simulink library "relay_housing_lib"  (Simulink 8.1)
settings: Solver=ode45  StartTime=0.0  StopTime=10.0  RelTol=1e-3
undefined symbols (not defined in the file): F0, F1, F2, F3, F4, Ts
libraries: relay_modbus_lib x137, rtio_generic_modbus x69, rtlab x10, simulink_extras x10, simulink x6, RMS_lib x4, relay_PLL_lib x3, powerlib_extras x2, relay_ANSI_functions_lib x2, relay_PQSPF_lib x1, powerlib_meascontrol x1, relay_mgc_cmd_lib x1
(part 1 of 3)
settings Model: Creator=re25624  LastModifiedBy=hptb1

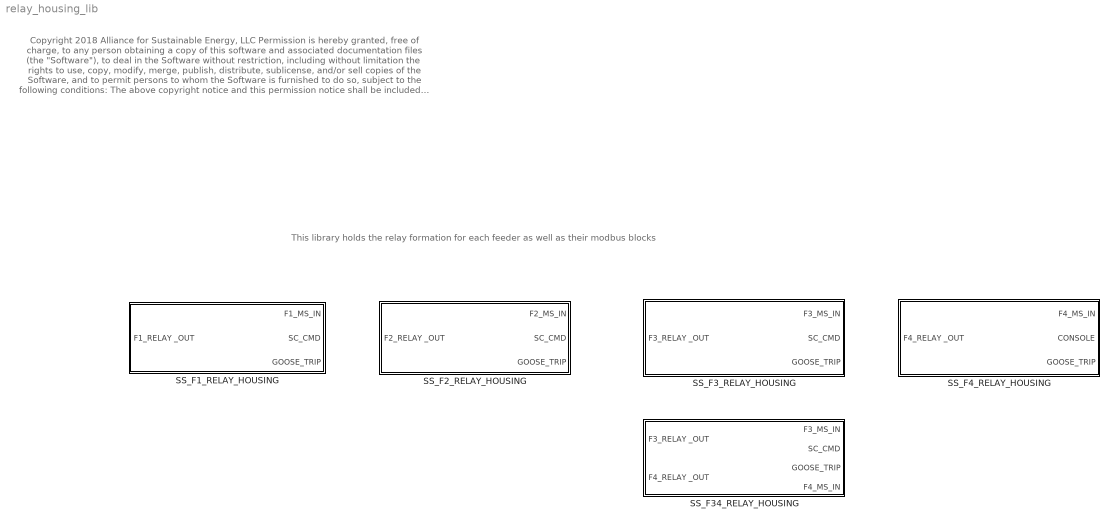
== system relay_housing_lib ==
  note: This library holds the relay formation for each feeder as well as their modbus blocks
  note: Copyright 2018 Alliance for Sustainable Energy, LLC
      |
      | Permission is hereby granted, free of charge, to any person obtaining a copy of this software
      | and associated documentation files (the "Software"), to deal in the Software without restriction,
      | including without limitation the rights to use, copy, modify, merge, publish, distribute, sublicense,
      | and/or sell copies of the Software, and to permit persons to whom the Software is furnished to do so,
      | subject to the following conditions:
      |
      | The above copyright notice and this permission notice shall be included in all copies or substantial portions of the Software.
      |
      | THE SOFTWARE IS PROVIDED "AS IS", WITHOUT WARRANTY OF ANY KIND, EXPRESS OR IMPLIED, INCLUDING
      | BUT NOT LIMITED TO THE WARRANTIES OF MERCHANTABILITY, FITNESS FOR A PARTICULAR PURPOSE AND
      | NONINFRINGEMENT. IN NO EVENT SHALL THE AUTHORS, THE COPYRIGHT HOLDERS, THE UNITED STATES,
      | THE UNITED STATES DEPARTMENT OF ENERGY, OR ANY OF THEIR EMPLOYEES BE LIABLE FOR ANY CLAIM,
      | DAMAGES OR OTHER LIABILITY, WHETHER IN AN ACTION OF CONTRACT, TORT OR OTHERWISE, ARISING FROM,
      | OUT OF OR IN CONNECTION WITH THE SOFTWARE OR THE USE OR OTHER DEALINGS IN THE SOFTWARE.
  SS_F1_RELAY_HOUSING : Subsystem
  SS_F2_RELAY_HOUSING : Subsystem
  SS_F34_RELAY_HOUSING : Subsystem
  SS_F3_RELAY_HOUSING : Subsystem
  SS_F4_RELAY_HOUSING : Subsystem

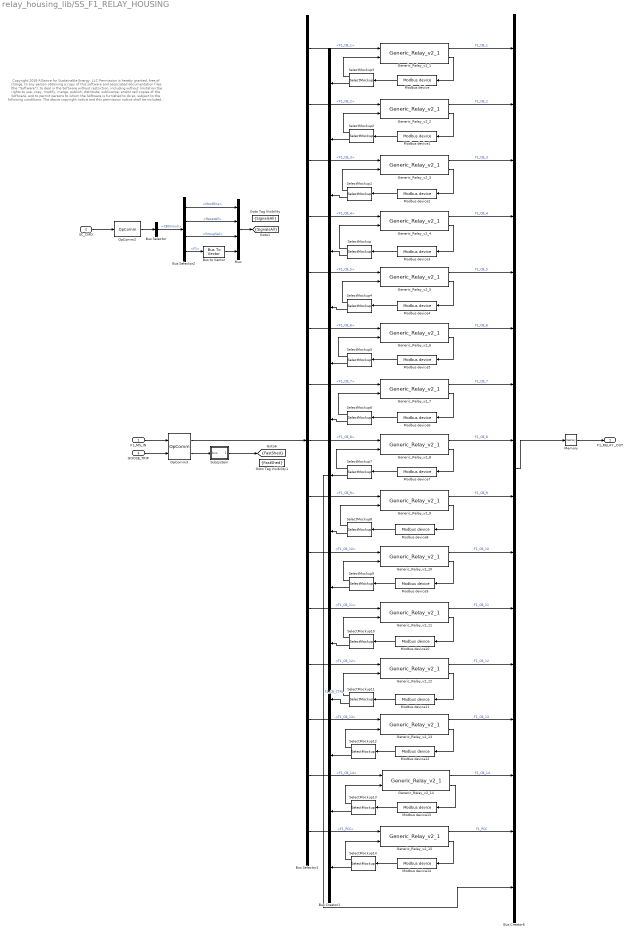
== system relay_housing_lib/SS_F1_RELAY_HOUSING ==
  note: Copyright 2018 Alliance for Sustainable Energy, LLC
      |
      | Permission is hereby granted, free of charge, to any person obtaining a copy of this software
      | and associated documentation files (the "Software"), to deal in the Software without restriction,
      | including without limitation the rights to use, copy, modify, merge, publish, distribute, sublicense,
      | and/or sell copies of the Software, and to permit persons to whom the Software is furnished to do so,
      | subject to the following conditions:
      |
      | The above copyright notice and this permission notice shall be included in all copies or substantial portions of the Software.
      |
      | THE SOFTWARE IS PROVIDED "AS IS", WITHOUT WARRANTY OF ANY KIND, EXPRESS OR IMPLIED, INCLUDING
      | BUT NOT LIMITED TO THE WARRANTIES OF MERCHANTABILITY, FITNESS FOR A PARTICULAR PURPOSE AND
      | NONINFRINGEMENT. IN NO EVENT SHALL THE AUTHORS, THE COPYRIGHT HOLDERS, THE UNITED STATES,
      | THE UNITED STATES DEPARTMENT OF ENERGY, OR ANY OF THEIR EMPLOYEES BE LIABLE FOR ANY CLAIM,
      | DAMAGES OR OTHER LIABILITY, WHETHER IN AN ACTION OF CONTRACT, TORT OR OTHERWISE, ARISING FROM,
      | OUT OF OR IN CONNECTION WITH THE SOFTWARE OR THE USE OR OTHER DEALINGS IN THE SOFTWARE.
  F1_MS_IN : Inport
  SC_CMD : Inport  Port=2
  GOOSE_TRIP : Inport  Port=3
  Bus Creator1 : BusCreator  Inputs=15
  Bus Creator6 : BusCreator  Inputs=16
  Bus Selector : BusSelector  OutputSignals=CBStimuli
  Bus Selector1 : BusSelector  OutputSignals=CB_DATA.F1_CB_1,CB_DATA.F1_CB_2,CB_DATA.F1_CB_3,CB_DATA.F1_CB_4,CB_DATA.F1_CB_5,CB_DATA.F1_CB_6,CB_DATA.F1_CB_7,CB_DATA.F1_CB_8,CB_DATA.F1_CB_9,CB_DATA.F1_CB_10,CB_DATA.F1_CB_11,CB_DATA.F1_CB_12,CB_DATA.F1_CB_13,CB_DATA.F1_CB_14,CB_DATA.F1_PCC
  Bus Selector2 : BusSelector  OutputSignals=MockEna,ResetAll,GroupSel,F1
  Bus to Vector : BusToVector
  Generic_Relay_v2_1 : relay_modbus_lib/Generic_Relay_v2_1  Ts=Ts  relay_settings=[F1(1,:)]
  Generic_Relay_v2_10 : relay_modbus_lib/Generic_Relay_v2_1  Ts=Ts  relay_settings=[F1(10,:)]
  Generic_Relay_v2_11 : relay_modbus_lib/Generic_Relay_v2_1  Ts=Ts  relay_settings=[F1(11,:)]
  Generic_Relay_v2_12 : relay_modbus_lib/Generic_Relay_v2_1  Ts=Ts  relay_settings=[F1(12,:)]
  Generic_Relay_v2_13 : relay_modbus_lib/Generic_Relay_v2_1  Ts=Ts  relay_settings=[F1(13,:)]
  Generic_Relay_v2_14 : relay_modbus_lib/Generic_Relay_v2_1  Ts=Ts  relay_settings=[F1(14,:)]
  Generic_Relay_v2_15 : relay_modbus_lib/Generic_Relay_v2_1  Ts=Ts  relay_settings=[F0(1,:)]
  Generic_Relay_v2_2 : relay_modbus_lib/Generic_Relay_v2_1  Ts=Ts  relay_settings=[F1(2,:)]
  Generic_Relay_v2_3 : relay_modbus_lib/Generic_Relay_v2_1  Ts=Ts  relay_settings=[F1(3,:)]
  Generic_Relay_v2_4 : relay_modbus_lib/Generic_Relay_v2_1  Ts=Ts  relay_settings=[F1(4,:)]
  Generic_Relay_v2_5 : relay_modbus_lib/Generic_Relay_v2_1  Ts=Ts  relay_settings=[F1(5,:)]
  Generic_Relay_v2_6 : relay_modbus_lib/Generic_Relay_v2_1  Ts=Ts  relay_settings=[F1(6,:)]
  Generic_Relay_v2_7 : relay_modbus_lib/Generic_Relay_v2_1  Ts=Ts  relay_settings=[F1(7,:)]
  Generic_Relay_v2_8 : relay_modbus_lib/Generic_Relay_v2_1  Ts=Ts  relay_settings=[F1(8,:)]
  Generic_Relay_v2_9 : relay_modbus_lib/Generic_Relay_v2_1  Ts=Ts  relay_settings=[F1(9,:)]
  Goto Tag Visibility : GotoTagVisibility  GotoTag=SignalsAll
  Goto Tag Visibility1 : GotoTagVisibility  GotoTag=FastShed
  Memory : Memory
  Modbus device : rtio_generic_modbus/Modbus device  conf_name=F1_relay_cfg1.opal  conf_name_mask=F1_relay_cfg1.xls  sample_time=Ts
  Modbus device1 : rtio_generic_modbus/Modbus device  conf_name=F1_relay_cfg2.opal  conf_name_mask=F1_relay_cfg2.xls  sample_time=Ts
  Modbus device10 : rtio_generic_modbus/Modbus device  conf_name=F1_relay_cfg11.opal  conf_name_mask=F1_relay_cfg11.xls  sample_time=Ts
  Modbus device11 : rtio_generic_modbus/Modbus device  conf_name=F1_relay_cfg12.opal  conf_name_mask=F1_relay_cfg12.xls  sample_time=Ts
  Modbus device12 : rtio_generic_modbus/Modbus device  conf_name=F1_relay_cfg13.opal  conf_name_mask=F1_relay_cfg13.xls  sample_time=Ts
  Modbus device13 : rtio_generic_modbus/Modbus device  conf_name=F1_relay_cfg14.opal  conf_name_mask=F1_relay_cfg14.xls  sample_time=Ts
  Modbus device14 : rtio_generic_modbus/Modbus device  conf_name=F1_relay_cfg_pcc.opal  conf_name_mask=F1_relay_cfg_pcc.xls  sample_time=Ts
  Modbus device2 : rtio_generic_modbus/Modbus device  conf_name=F1_relay_cfg3.opal  conf_name_mask=F1_relay_cfg3.xls  sample_time=Ts
  Modbus device3 : rtio_generic_modbus/Modbus device  conf_name=F1_relay_cfg4.opal  conf_name_mask=F1_relay_cfg4.xls  sample_time=Ts
  Modbus device4 : rtio_generic_modbus/Modbus device  conf_name=F1_relay_cfg5.opal  conf_name_mask=F1_relay_cfg5.xls  sample_time=Ts
  Modbus device5 : rtio_generic_modbus/Modbus device  conf_name=F1_relay_cfg6.opal  conf_name_mask=F1_relay_cfg6.xls  sample_time=Ts
  Modbus device6 : rtio_generic_modbus/Modbus device  conf_name=F1_relay_cfg7.opal  conf_name_mask=F1_relay_cfg7.xls  sample_time=Ts
  Modbus device7 : rtio_generic_modbus/Modbus device  conf_name=F1_relay_cfg8.opal  conf_name_mask=F1_relay_cfg8.xls  sample_time=Ts
  Modbus device8 : rtio_generic_modbus/Modbus device  conf_name=F1_relay_cfg9.opal  conf_name_mask=F1_relay_cfg9.xls  sample_time=Ts
  Modbus device9 : rtio_generic_modbus/Modbus device  conf_name=F1_relay_cfg10.opal  conf_name_mask=F1_relay_cfg10.xls  sample_time=Ts
  Mux : Mux
  OpComm2 : rtlab/OpComm  nbport=1  groupe_acq=1  subsys_rate=0  st=0  Synchronization=on  Interpolation=on  Threshold=1.0  Missed_Data=off  Sim_Time=off  Samples=off  dynSigOut=off  from_console=1  warning_done=off  writeOpCommFile=off  Offset=off
  OpComm3 : rtlab/OpComm  nbport=2  groupe_acq=1  subsys_rate=0  st=0  Synchronization=on  Interpolation=on  Threshold=1.0  Missed_Data=off  Sim_Time=off  Samples=off  dynSigOut=off  from_console=0  warning_done=off  writeOpCommFile=off  Offset=off
  SelectMockup : relay_modbus_lib/SelectMockup  sigID=4  sigN=15
  SelectMockup1 : relay_modbus_lib/SelectMockup  sigID=3  sigN=15
  SelectMockup10 : relay_modbus_lib/SelectMockup  sigID=11  sigN=15
  SelectMockup11 : relay_modbus_lib/SelectMockup  sigID=12  sigN=15
  SelectMockup12 : relay_modbus_lib/SelectMockup  sigID=13  sigN=15
  SelectMockup13 : relay_modbus_lib/SelectMockup  sigID=14  sigN=15
  SelectMockup14 : relay_modbus_lib/SelectMockup  sigID=15  sigN=15
  SelectMockup2 : relay_modbus_lib/SelectMockup  sigID=2  sigN=15
  SelectMockup3 : relay_modbus_lib/SelectMockup  sigID=1  sigN=15
  SelectMockup4 : relay_modbus_lib/SelectMockup  sigID=5  sigN=15
  SelectMockup5 : relay_modbus_lib/SelectMockup  sigID=6  sigN=15
  SelectMockup6 : relay_modbus_lib/SelectMockup  sigID=7  sigN=15
  SelectMockup7 : relay_modbus_lib/SelectMockup  sigID=8  sigN=15
  SelectMockup8 : relay_modbus_lib/SelectMockup  sigID=9  sigN=15
  SelectMockup9 : relay_modbus_lib/SelectMockup  sigID=10  sigN=15
  Subsystem : Subsystem
  F1_RELAY _OUT : Outport
  tag scope: FastShed=scoped, SignalsAll=scoped
  wires:
  SelectMockup14/2 -> Bus Creator1/15
  SelectMockup13/2 -> Bus Creator1/14
  SelectMockup12/2 -> Bus Creator1/13
  SelectMockup11/2 -> Bus Creator1/12
  SelectMockup10/2 -> Bus Creator1/11
  SelectMockup9/2 -> Bus Creator1/10
  Bus Creator1/1 -> Bus Creator6/16  "F1_CB_CTRL"
  SelectMockup8/2 -> Bus Creator1/9
  SelectMockup7/2 -> Bus Creator1/8
  SelectMockup6/2 -> Bus Creator1/7
  SelectMockup5/2 -> Bus Creator1/6
  SelectMockup4/2 -> Bus Creator1/5
  SelectMockup/2 -> Bus Creator1/4
  SelectMockup1/2 -> Bus Creator1/3
  SelectMockup2/2 -> Bus Creator1/2
  SelectMockup3/2 -> Bus Creator1/1
  OpComm3/2 -> Subsystem/1(bus)
  Subsystem/1(vect) -> [FastShed]
  GOOSE_TRIP/1 -> OpComm3/2
  SelectMockup13/1 -> Generic_Relay_v2_14/2
  Modbus device13/1 -> SelectMockup13/1
  SelectMockup14/1 -> Generic_Relay_v2_15/2
  Modbus device14/1 -> SelectMockup14/1
  SelectMockup12/1 -> Generic_Relay_v2_13/2
  Modbus device12/1 -> SelectMockup12/1
  SelectMockup11/1 -> Generic_Relay_v2_12/2
  Modbus device11/1 -> SelectMockup11/1
  SelectMockup10/1 -> Generic_Relay_v2_11/2
  Modbus device10/1 -> SelectMockup10/1
  SelectMockup9/1 -> Generic_Relay_v2_10/2
  Modbus device9/1 -> SelectMockup9/1
  SelectMockup8/1 -> Generic_Relay_v2_9/2
  Modbus device8/1 -> SelectMockup8/1
  SelectMockup7/1 -> Generic_Relay_v2_8/2
  Modbus device7/1 -> SelectMockup7/1
  SelectMockup6/1 -> Generic_Relay_v2_7/2
  Modbus device6/1 -> SelectMockup6/1
  SelectMockup5/1 -> Generic_Relay_v2_6/2
  Modbus device5/1 -> SelectMockup5/1
  SelectMockup4/1 -> Generic_Relay_v2_5/2
  Modbus device4/1 -> SelectMockup4/1
  Modbus device/1 -> SelectMockup3/1
  Modbus device1/1 -> SelectMockup2/1
  Modbus device2/1 -> SelectMockup1/1
  Modbus device3/1 -> SelectMockup/1
  Mux/1 -> [SignalsAll]
  Bus Selector2/2 -> Mux/2  "<ResetAll>"
  Bus Selector2/3 -> Mux/3  "<GroupSel>"
  Bus to Vector/1 -> Mux/4
  SelectMockup3/1 -> Generic_Relay_v2_1/2
  SelectMockup2/1 -> Generic_Relay_v2_2/2
  Bus Selector2/1 -> Mux/1  "<MockEna>"
  SelectMockup1/1 -> Generic_Relay_v2_3/2
  SelectMockup/1 -> Generic_Relay_v2_4/2
  Bus Selector2/4 -> Bus to Vector/1  "<F1>"
  Bus Selector/1 -> Bus Selector2/1  "<CBStimuli>"
  OpComm2/1 -> Bus Selector/1
  SC_CMD/1 -> OpComm2/1
  Generic_Relay_v2_15/1 -> Bus Creator6/15  "F1_PCC"
  Bus Selector1/15 -> Generic_Relay_v2_15/1  "<F1_PCC>"
  Generic_Relay_v2_15/2 -> Modbus device14/1
  Memory/1 -> F1_RELAY _OUT/1
  Bus Selector1/14 -> Generic_Relay_v2_14/1  "<F1_CB_14>"
  Generic_Relay_v2_14/1 -> Bus Creator6/14  "F1_CB_14"
  Generic_Relay_v2_14/2 -> Modbus device13/1
  Generic_Relay_v2_3/1 -> Bus Creator6/3  "F1_CB_3"
  Generic_Relay_v2_4/1 -> Bus Creator6/4  "F1_CB_4"
  Generic_Relay_v2_5/1 -> Bus Creator6/5  "F1_CB_5"
  Generic_Relay_v2_6/1 -> Bus Creator6/6  "F1_CB_6"
  Generic_Relay_v2_7/1 -> Bus Creator6/7  "F1_CB_7"
  Generic_Relay_v2_8/1 -> Bus Creator6/8  "F1_CB_8"
  Generic_Relay_v2_9/1 -> Bus Creator6/9  "F1_CB_9"
  Generic_Relay_v2_10/1 -> Bus Creator6/10  "F1_CB_10"
  Generic_Relay_v2_11/1 -> Bus Creator6/11  "F1_CB_11"
  Generic_Relay_v2_12/1 -> Bus Creator6/12  "F1_CB_12"
  Generic_Relay_v2_13/1 -> Bus Creator6/13  "F1_CB_13"
  Bus Selector1/13 -> Generic_Relay_v2_13/1  "<F1_CB_13>"
  Bus Selector1/12 -> Generic_Relay_v2_12/1  "<F1_CB_12>"
  Bus Selector1/11 -> Generic_Relay_v2_11/1  "<F1_CB_11>"
  Bus Selector1/10 -> Generic_Relay_v2_10/1  "<F1_CB_10>"
  Bus Selector1/9 -> Generic_Relay_v2_9/1  "<F1_CB_9>"
  Bus Selector1/8 -> Generic_Relay_v2_8/1  "<F1_CB_8>"
  Bus Selector1/7 -> Generic_Relay_v2_7/1  "<F1_CB_7>"
  Bus Selector1/6 -> Generic_Relay_v2_6/1  "<F1_CB_6>"
  Bus Selector1/5 -> Generic_Relay_v2_5/1  "<F1_CB_5>"
  Bus Selector1/4 -> Generic_Relay_v2_4/1  "<F1_CB_4>"
  Bus Selector1/3 -> Generic_Relay_v2_3/1  "<F1_CB_3>"
  Generic_Relay_v2_2/1 -> Bus Creator6/2  "F1_CB_2"
  Bus Selector1/2 -> Generic_Relay_v2_2/1  "<F1_CB_2>"
  Bus Creator6/1 -> Memory/1
  Generic_Relay_v2_1/1 -> Bus Creator6/1  "F1_CB_1"
  Bus Selector1/1 -> Generic_Relay_v2_1/1  "<F1_CB_1>"
  F1_MS_IN/1 -> OpComm3/1
  Generic_Relay_v2_1/2 -> Modbus device/1
  Generic_Relay_v2_2/2 -> Modbus device1/1
  Generic_Relay_v2_3/2 -> Modbus device2/1
  Generic_Relay_v2_4/2 -> Modbus device3/1
  Generic_Relay_v2_5/2 -> Modbus device4/1
  Generic_Relay_v2_6/2 -> Modbus device5/1
  Generic_Relay_v2_7/2 -> Modbus device6/1
  Generic_Relay_v2_8/2 -> Modbus device7/1
  Generic_Relay_v2_9/2 -> Modbus device8/1
  Generic_Relay_v2_10/2 -> Modbus device9/1
  Generic_Relay_v2_11/2 -> Modbus device10/1
  Generic_Relay_v2_12/2 -> Modbus device11/1
  Generic_Relay_v2_13/2 -> Modbus device12/1
  OpComm3/1 -> Bus Selector1/1

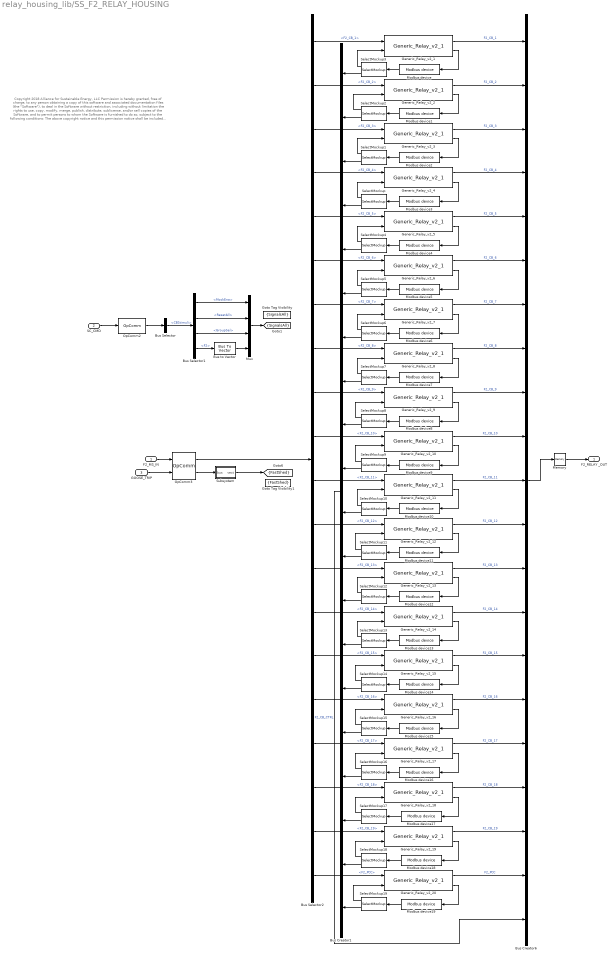
== system relay_housing_lib/SS_F2_RELAY_HOUSING ==
  note: Copyright 2018 Alliance for Sustainable Energy, LLC
      |
      | Permission is hereby granted, free of charge, to any person obtaining a copy of this software
      | and associated documentation files (the "Software"), to deal in the Software without restriction,
      | including without limitation the rights to use, copy, modify, merge, publish, distribute, sublicense,
      | and/or sell copies of the Software, and to permit persons to whom the Software is furnished to do so,
      | subject to the following conditions:
      |
      | The above copyright notice and this permission notice shall be included in all copies or substantial portions of the Software.
      |
      | THE SOFTWARE IS PROVIDED "AS IS", WITHOUT WARRANTY OF ANY KIND, EXPRESS OR IMPLIED, INCLUDING
      | BUT NOT LIMITED TO THE WARRANTIES OF MERCHANTABILITY, FITNESS FOR A PARTICULAR PURPOSE AND
      | NONINFRINGEMENT. IN NO EVENT SHALL THE AUTHORS, THE COPYRIGHT HOLDERS, THE UNITED STATES,
      | THE UNITED STATES DEPARTMENT OF ENERGY, OR ANY OF THEIR EMPLOYEES BE LIABLE FOR ANY CLAIM,
      | DAMAGES OR OTHER LIABILITY, WHETHER IN AN ACTION OF CONTRACT, TORT OR OTHERWISE, ARISING FROM,
      | OUT OF OR IN CONNECTION WITH THE SOFTWARE OR THE USE OR OTHER DEALINGS IN THE SOFTWARE.
  F2_MS_IN : Inport
  SC_CMD : Inport  Port=2
  GOOSE_TRIP : Inport  Port=3
  Bus Creator1 : BusCreator  Inputs=20
  Bus Creator6 : BusCreator  Inputs=21
  Bus Selector : BusSelector  OutputSignals=CBStimuli
  Bus Selector1 : BusSelector  OutputSignals=MockEna,ResetAll,GroupSel,F2
  Bus Selector2 : BusSelector  OutputSignals=CB_DATA.F2_CB_1,CB_DATA.F2_CB_2,CB_DATA.F2_CB_3,CB_DATA.F2_CB_4,CB_DATA.F2_CB_5,CB_DATA.F2_CB_6,CB_DATA.F2_CB_7,CB_DATA.F2_CB_8,CB_DATA.F2_CB_9,CB_DATA.F2_CB_10,CB_DATA.F2_CB_11,CB_DATA.F2_CB_12,CB_DATA.F2_CB_13,CB_DATA.F2_CB_14,CB_DATA.F2_CB_15,CB_DATA.F2_CB_16,CB_DATA.F2_CB_17,CB_DATA.F2_CB_18,CB_DATA.F2_CB_19,CB_DATA.F2_PCC
  Bus to Vector : BusToVector
  Generic_Relay_v2_1 : relay_modbus_lib/Generic_Relay_v2_1  Ts=Ts  relay_settings=[F2(1,:)]
  Generic_Relay_v2_10 : relay_modbus_lib/Generic_Relay_v2_1  Ts=Ts  relay_settings=[F2(10,:)]
  Generic_Relay_v2_11 : relay_modbus_lib/Generic_Relay_v2_1  Ts=Ts  relay_settings=[F2(11,:)]
  Generic_Relay_v2_12 : relay_modbus_lib/Generic_Relay_v2_1  Ts=Ts  relay_settings=[F2(12,:)]
  Generic_Relay_v2_13 : relay_modbus_lib/Generic_Relay_v2_1  Ts=Ts  relay_settings=[F2(13,:)]
  Generic_Relay_v2_14 : relay_modbus_lib/Generic_Relay_v2_1  Ts=Ts  relay_settings=[F2(14,:)]
  Generic_Relay_v2_15 : relay_modbus_lib/Generic_Relay_v2_1  Ts=Ts  relay_settings=[F2(15,:)]
  Generic_Relay_v2_16 : relay_modbus_lib/Generic_Relay_v2_1  Ts=Ts  relay_settings=[F2(16,:)]
  Generic_Relay_v2_17 : relay_modbus_lib/Generic_Relay_v2_1  Ts=Ts  relay_settings=[F2(17,:)]
  Generic_Relay_v2_18 : relay_modbus_lib/Generic_Relay_v2_1  Ts=Ts  relay_settings=[F2(18,:)]
  Generic_Relay_v2_19 : relay_modbus_lib/Generic_Relay_v2_1  Ts=Ts  relay_settings=[F2(19,:)]
  Generic_Relay_v2_2 : relay_modbus_lib/Generic_Relay_v2_1  Ts=Ts  relay_settings=[F2(2,:)]
  Generic_Relay_v2_20 : relay_modbus_lib/Generic_Relay_v2_1  Ts=Ts  relay_settings=[F0(2,:)]
  Generic_Relay_v2_3 : relay_modbus_lib/Generic_Relay_v2_1  Ts=Ts  relay_settings=[F2(3,:)]
  Generic_Relay_v2_4 : relay_modbus_lib/Generic_Relay_v2_1  Ts=Ts  relay_settings=[F2(4,:)]
  Generic_Relay_v2_5 : relay_modbus_lib/Generic_Relay_v2_1  Ts=Ts  relay_settings=[F2(5,:)]
  Generic_Relay_v2_6 : relay_modbus_lib/Generic_Relay_v2_1  Ts=Ts  relay_settings=[F2(6,:)]
  Generic_Relay_v2_7 : relay_modbus_lib/Generic_Relay_v2_1  Ts=Ts  relay_settings=[F2(7,:)]
  Generic_Relay_v2_8 : relay_modbus_lib/Generic_Relay_v2_1  Ts=Ts  relay_settings=[F2(8,:)]
  Generic_Relay_v2_9 : relay_modbus_lib/Generic_Relay_v2_1  Ts=Ts  relay_settings=[F2(9,:)]
  Goto Tag Visibility : GotoTagVisibility  GotoTag=SignalsAll
  Goto Tag Visibility1 : GotoTagVisibility  GotoTag=FastShed
  Memory : Memory
  Modbus device : rtio_generic_modbus/Modbus device  conf_name=F2_relay_cfg1.opal  conf_name_mask=F2_relay_cfg1.xls  sample_time=Ts
  Modbus device1 : rtio_generic_modbus/Modbus device  conf_name=F2_relay_cfg2.opal  conf_name_mask=F2_relay_cfg2.xls  sample_time=Ts
  Modbus device10 : rtio_generic_modbus/Modbus device  conf_name=F2_relay_cfg11.opal  conf_name_mask=F2_relay_cfg11.xls  sample_time=Ts
  Modbus device11 : rtio_generic_modbus/Modbus device  conf_name=F2_relay_cfg12.opal  conf_name_mask=F2_relay_cfg12.xls  sample_time=Ts
  Modbus device12 : rtio_generic_modbus/Modbus device  conf_name=F2_relay_cfg13.opal  conf_name_mask=F2_relay_cfg13.xls  sample_time=Ts
  Modbus device13 : rtio_generic_modbus/Modbus device  conf_name=F2_relay_cfg14.opal  conf_name_mask=F2_relay_cfg14.xls  sample_time=Ts
  Modbus device14 : rtio_generic_modbus/Modbus device  conf_name=F2_relay_cfg15.opal  conf_name_mask=F2_relay_cfg15.xls  sample_time=Ts
  Modbus device15 : rtio_generic_modbus/Modbus device  conf_name=F2_relay_cfg16.opal  conf_name_mask=F2_relay_cfg16.xls  sample_time=Ts
  Modbus device16 : rtio_generic_modbus/Modbus device  conf_name=F2_relay_cfg17.opal  conf_name_mask=F2_relay_cfg17.xls  sample_time=Ts
  Modbus device17 : rtio_generic_modbus/Modbus device  conf_name=F2_relay_cfg18.opal  conf_name_mask=F2_relay_cfg18.xls  sample_time=Ts
  Modbus device18 : rtio_generic_modbus/Modbus device  conf_name=F2_relay_cfg19.opal  conf_name_mask=F2_relay_cfg19.xls  sample_time=Ts
  Modbus device19 : rtio_generic_modbus/Modbus device  conf_name=F2_relay_cfg_pcc.opal  conf_name_mask=F2_relay_cfg_pcc.xls  sample_time=Ts
  Modbus device2 : rtio_generic_modbus/Modbus device  conf_name=F2_relay_cfg3.opal  conf_name_mask=F2_relay_cfg3.xls  sample_time=Ts
  Modbus device3 : rtio_generic_modbus/Modbus device  conf_name=F2_relay_cfg4.opal  conf_name_mask=F2_relay_cfg4.xls  sample_time=Ts
  Modbus device4 : rtio_generic_modbus/Modbus device  conf_name=F2_relay_cfg5.opal  conf_name_mask=F2_relay_cfg5.xls  sample_time=Ts
  Modbus device5 : rtio_generic_modbus/Modbus device  conf_name=F2_relay_cfg6.opal  conf_name_mask=F2_relay_cfg6.xls  sample_time=Ts
  Modbus device6 : rtio_generic_modbus/Modbus device  conf_name=F2_relay_cfg7.opal  conf_name_mask=F2_relay_cfg7.xls  sample_time=Ts
  Modbus device7 : rtio_generic_modbus/Modbus device  conf_name=F2_relay_cfg8.opal  conf_name_mask=F2_relay_cfg8.xls  sample_time=Ts
  Modbus device8 : rtio_generic_modbus/Modbus device  conf_name=F2_relay_cfg9.opal  conf_name_mask=F2_relay_cfg9.xls  sample_time=Ts
  Modbus device9 : rtio_generic_modbus/Modbus device  conf_name=F2_relay_cfg10.opal  conf_name_mask=F2_relay_cfg10.xls  sample_time=Ts
  Mux : Mux
  OpComm2 : rtlab/OpComm  nbport=1  groupe_acq=1  subsys_rate=0  st=0  Synchronization=on  Interpolation=on  Threshold=1.0  Missed_Data=off  Sim_Time=off  Samples=off  dynSigOut=off  from_console=1  warning_done=off  writeOpCommFile=off  Offset=off
  OpComm3 : rtlab/OpComm  nbport=2  groupe_acq=1  subsys_rate=0  st=0  Synchronization=on  Interpolation=on  Threshold=1.0  Missed_Data=off  Sim_Time=off  Samples=off  dynSigOut=off  from_console=0  warning_done=off  writeOpCommFile=off  Offset=off
  SelectMockup : relay_modbus_lib/SelectMockup  sigID=4  sigN=20
  SelectMockup1 : relay_modbus_lib/SelectMockup  sigID=3  sigN=20
  SelectMockup10 : relay_modbus_lib/SelectMockup  sigID=11  sigN=20
  SelectMockup11 : relay_modbus_lib/SelectMockup  sigID=12  sigN=20
  SelectMockup12 : relay_modbus_lib/SelectMockup  sigID=13  sigN=20
  SelectMockup13 : relay_modbus_lib/SelectMockup  sigID=14  sigN=20
  SelectMockup14 : relay_modbus_lib/SelectMockup  sigID=15  sigN=20
  SelectMockup15 : relay_modbus_lib/SelectMockup  sigID=16  sigN=20
  SelectMockup16 : relay_modbus_lib/SelectMockup  sigID=17  sigN=20
  SelectMockup17 : relay_modbus_lib/SelectMockup  sigID=18  sigN=20
  SelectMockup18 : relay_modbus_lib/SelectMockup  sigID=19  sigN=20
  SelectMockup19 : relay_modbus_lib/SelectMockup  sigID=20  sigN=20
  SelectMockup2 : relay_modbus_lib/SelectMockup  sigID=2  sigN=20
  SelectMockup3 : relay_modbus_lib/SelectMockup  sigID=1  sigN=20
  SelectMockup4 : relay_modbus_lib/SelectMockup  sigID=5  sigN=20
  SelectMockup5 : relay_modbus_lib/SelectMockup  sigID=6  sigN=20
  SelectMockup6 : relay_modbus_lib/SelectMockup  sigID=7  sigN=20
  SelectMockup7 : relay_modbus_lib/SelectMockup  sigID=8  sigN=20
  SelectMockup8 : relay_modbus_lib/SelectMockup  sigID=9  sigN=20
  SelectMockup9 : relay_modbus_lib/SelectMockup  sigID=10  sigN=20
  Subsystem : Subsystem
  F2_RELAY _OUT : Outport
  tag scope: FastShed=scoped, SignalsAll=scoped
  wires:
  SelectMockup19/2 -> Bus Creator1/20
  SelectMockup18/2 -> Bus Creator1/19
  SelectMockup17/2 -> Bus Creator1/18
  SelectMockup16/2 -> Bus Creator1/17
  SelectMockup15/2 -> Bus Creator1/16
  SelectMockup14/2 -> Bus Creator1/15
  SelectMockup13/2 -> Bus Creator1/14
  SelectMockup12/2 -> Bus Creator1/13
  SelectMockup11/2 -> Bus Creator1/12
  SelectMockup10/2 -> Bus Creator1/11
  Bus Creator1/1 -> Bus Creator6/21  "F2_CB_CTRL"
  SelectMockup9/2 -> Bus Creator1/10
  SelectMockup8/2 -> Bus Creator1/9
  SelectMockup7/2 -> Bus Creator1/8
  SelectMockup6/2 -> Bus Creator1/7
  SelectMockup5/2 -> Bus Creator1/6
  SelectMockup4/2 -> Bus Creator1/5
  SelectMockup/2 -> Bus Creator1/4
  SelectMockup1/2 -> Bus Creator1/3
  SelectMockup2/2 -> Bus Creator1/2
  SelectMockup3/2 -> Bus Creator1/1
  Subsystem/1(vect) -> [FastShed]
  OpComm3/2 -> Subsystem/1(bus)
  GOOSE_TRIP/1 -> OpComm3/2
  Mux/1 -> [SignalsAll]
  Bus Selector1/2 -> Mux/2  "<ResetAll>"
  Bus Selector1/3 -> Mux/3  "<GroupSel>"
  Bus to Vector/1 -> Mux/4
  Bus Selector1/1 -> Mux/1  "<MockEna>"
  Bus Selector1/4 -> Bus to Vector/1  "<F2>"
  Bus Selector/1 -> Bus Selector1/1  "<CBStimuli>"
  OpComm2/1 -> Bus Selector/1
  SC_CMD/1 -> OpComm2/1
  Modbus device19/1 -> SelectMockup19/1
  Modbus device/1 -> SelectMockup3/1
  Modbus device1/1 -> SelectMockup2/1
  Modbus device2/1 -> SelectMockup1/1
  Modbus device3/1 -> SelectMockup/1
  Modbus device4/1 -> SelectMockup4/1
  Modbus device5/1 -> SelectMockup5/1
  Modbus device6/1 -> SelectMockup6/1
  Modbus device7/1 -> SelectMockup7/1
  Modbus device8/1 -> SelectMockup8/1
  Modbus device9/1 -> SelectMockup9/1
  Modbus device10/1 -> SelectMockup10/1
  Modbus device11/1 -> SelectMockup11/1
  Modbus device12/1 -> SelectMockup12/1
  Modbus device13/1 -> SelectMockup13/1
  Modbus device14/1 -> SelectMockup14/1
  Modbus device15/1 -> SelectMockup15/1
  Modbus device16/1 -> SelectMockup16/1
  Modbus device17/1 -> SelectMockup17/1
  Modbus device18/1 -> SelectMockup18/1
  Bus Selector2/20 -> Generic_Relay_v2_20/1  "<F2_PCC>"
  Generic_Relay_v2_20/1 -> Bus Creator6/20  "F2_PCC"
  Generic_Relay_v2_20/2 -> Modbus device19/1
  SelectMockup19/1 -> Generic_Relay_v2_20/2
  Memory/1 -> F2_RELAY _OUT/1
  Bus Selector2/18 -> Generic_Relay_v2_18/1  "<F2_CB_18>"
  Bus Selector2/19 -> Generic_Relay_v2_19/1  "<F2_CB_19>"
  Generic_Relay_v2_19/1 -> Bus Creator6/19  "F2_CB_19"
  Generic_Relay_v2_18/1 -> Bus Creator6/18  "F2_CB_18"
  Generic_Relay_v2_18/2 -> Modbus device17/1
  SelectMockup17/1 -> Generic_Relay_v2_18/2
  Generic_Relay_v2_19/2 -> Modbus device18/1
  SelectMockup18/1 -> Generic_Relay_v2_19/2
  Bus Selector2/17 -> Generic_Relay_v2_17/1  "<F2_CB_17>"
  Generic_Relay_v2_17/1 -> Bus Creator6/17  "F2_CB_17"
  Generic_Relay_v2_6/1 -> Bus Creator6/6  "F2_CB_6"
  Generic_Relay_v2_5/1 -> Bus Creator6/5  "F2_CB_5"
  Generic_Relay_v2_4/1 -> Bus Creator6/4  "F2_CB_4"
  Generic_Relay_v2_3/1 -> Bus Creator6/3  "F2_CB_3"
  Generic_Relay_v2_2/1 -> Bus Creator6/2  "F2_CB_2"
  Generic_Relay_v2_7/1 -> Bus Creator6/7  "F2_CB_7"
  Generic_Relay_v2_8/1 -> Bus Creator6/8  "F2_CB_8"
  Generic_Relay_v2_9/1 -> Bus Creator6/9  "F2_CB_9"
  Generic_Relay_v2_10/1 -> Bus Creator6/10  "F2_CB_10"
  Generic_Relay_v2_11/1 -> Bus Creator6/11  "F2_CB_11"
  Generic_Relay_v2_16/1 -> Bus Creator6/16  "F2_CB_16"
  Generic_Relay_v2_15/1 -> Bus Creator6/15  "F2_CB_15"
  Generic_Relay_v2_14/1 -> Bus Creator6/14  "F2_CB_14"
  Generic_Relay_v2_13/1 -> Bus Creator6/13  "F2_CB_13"
  Generic_Relay_v2_12/1 -> Bus Creator6/12  "F2_CB_12"
  Bus Selector2/16 -> Generic_Relay_v2_16/1  "<F2_CB_16>"
  Bus Selector2/15 -> Generic_Relay_v2_15/1  "<F2_CB_15>"
  Bus Selector2/14 -> Generic_Relay_v2_14/1  "<F2_CB_14>"
  Bus Selector2/13 -> Generic_Relay_v2_13/1  "<F2_CB_13>"
  Bus Selector2/12 -> Generic_Relay_v2_12/1  "<F2_CB_12>"
  Bus Selector2/11 -> Generic_Relay_v2_11/1  "<F2_CB_11>"
  Bus Selector2/10 -> Generic_Relay_v2_10/1  "<F2_CB_10>"
  Bus Selector2/9 -> Generic_Relay_v2_9/1  "<F2_CB_9>"
  Bus Selector2/8 -> Generic_Relay_v2_8/1  "<F2_CB_8>"
  Bus Selector2/7 -> Generic_Relay_v2_7/1  "<F2_CB_7>"
  Bus Selector2/6 -> Generic_Relay_v2_6/1  "<F2_CB_6>"
  Bus Selector2/5 -> Generic_Relay_v2_5/1  "<F2_CB_5>"
  Bus Selector2/4 -> Generic_Relay_v2_4/1  "<F2_CB_4>"
  Bus Selector2/3 -> Generic_Relay_v2_3/1  "<F2_CB_3>"
  Bus Selector2/2 -> Generic_Relay_v2_2/1  "<F2_CB_2>"
  Generic_Relay_v2_1/1 -> Bus Creator6/1  "F2_CB_1"
  Bus Selector2/1 -> Generic_Relay_v2_1/1  "<F2_CB_1>"
  F2_MS_IN/1 -> OpComm3/1
  Bus Creator6/1 -> Memory/1
  Generic_Relay_v2_1/2 -> Modbus device/1
  SelectMockup3/1 -> Generic_Relay_v2_1/2
  Generic_Relay_v2_2/2 -> Modbus device1/1
  SelectMockup2/1 -> Generic_Relay_v2_2/2
  Generic_Relay_v2_3/2 -> Modbus device2/1
  SelectMockup1/1 -> Generic_Relay_v2_3/2
  Generic_Relay_v2_4/2 -> Modbus device3/1
  SelectMockup/1 -> Generic_Relay_v2_4/2
  Generic_Relay_v2_5/2 -> Modbus device4/1
  SelectMockup4/1 -> Generic_Relay_v2_5/2
  SelectMockup5/1 -> Generic_Relay_v2_6/2
  Generic_Relay_v2_6/2 -> Modbus device5/1
  Generic_Relay_v2_7/2 -> Modbus device6/1
  SelectMockup6/1 -> Generic_Relay_v2_7/2
  Generic_Relay_v2_8/2 -> Modbus device7/1
  SelectMockup7/1 -> Generic_Relay_v2_8/2
  Generic_Relay_v2_9/2 -> Modbus device8/1
  SelectMockup8/1 -> Generic_Relay_v2_9/2
  Generic_Relay_v2_10/2 -> Modbus device9/1
  SelectMockup9/1 -> Generic_Relay_v2_10/2
  Generic_Relay_v2_11/2 -> Modbus device10/1
  SelectMockup10/1 -> Generic_Relay_v2_11/2
  Generic_Relay_v2_12/2 -> Modbus device11/1
  SelectMockup11/1 -> Generic_Relay_v2_12/2
  SelectMockup12/1 -> Generic_Relay_v2_13/2
  Generic_Relay_v2_13/2 -> Modbus device12/1
  Generic_Relay_v2_14/2 -> Modbus device13/1
  SelectMockup13/1 -> Generic_Relay_v2_14/2
  Generic_Relay_v2_15/2 -> Modbus device14/1
  SelectMockup14/1 -> Generic_Relay_v2_15/2
  Generic_Relay_v2_16/2 -> Modbus device15/1
  SelectMockup15/1 -> Generic_Relay_v2_16/2
  Generic_Relay_v2_17/2 -> Modbus device16/1
  SelectMockup16/1 -> Generic_Relay_v2_17/2
  OpComm3/1 -> Bus Selector2/1

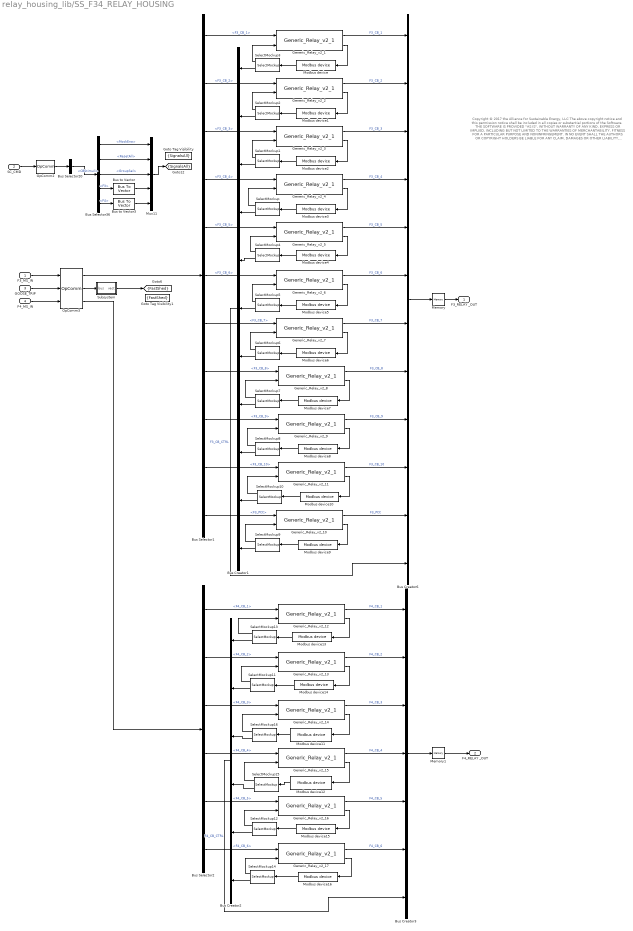
== system relay_housing_lib/SS_F34_RELAY_HOUSING ==
  note: Copyright © 2017 the Alliance for Sustainable Energy, LLC
      |
      | The above copyright notice and this permission notice shall be included in all copies or substantial portions of the Software.
      |
      | THE SOFTWARE IS PROVIDED "AS IS", WITHOUT WARRANTY OF ANY KIND, EXPRESS OR IMPLIED, INCLUDING
      | BUT NOT LIMITED TO THE WARRANTIES OF MERCHANTABILITY, FITNESS FOR A PARTICULAR PURPOSE AND
      | NONINFRINGEMENT. IN NO EVENT SHALL THE AUTHORS OR COPYRIGHT HOLDERS BE LIABLE FOR ANY CLAIM,
      |  DAMAGES OR OTHER LIABILITY, WHETHER IN AN ACTION OF CONTRACT, TORT OR OTHERWISE, ARISING FROM,
      | OUT OF OR IN CONNECTION WITH THE SOFTWARE OR THE USE OR OTHER DEALINGS IN THE SOFTWARE
  F3_MS_IN : Inport
  SC_CMD : Inport  Port=2
  GOOSE_TRIP : Inport  Port=3
  F4_MS_IN : Inport  Port=4
  Bus Creator1 : BusCreator  Inputs=11
  Bus Creator2 : BusCreator  Inputs=6
  Bus Creator3 : BusCreator  Inputs=7
  Bus Creator6 : BusCreator  Inputs=12
  Bus Selector1 : BusSelector  OutputSignals=CB_DATA.F3_CB_1,CB_DATA.F3_CB_2,CB_DATA.F3_CB_3,CB_DATA.F3_CB_4,CB_DATA.F3_CB_5,CB_DATA.F3_CB_6,CB_DATA.F3_CB_7,CB_DATA.F3_CB_8,CB_DATA.F3_CB_9,CB_DATA.F3_CB_10,CB_DATA.F3_PCC
  Bus Selector2 : BusSelector  OutputSignals=CB_DATA.F4_CB_1,CB_DATA.F4_CB_2,CB_DATA.F4_CB_3,CB_DATA.F4_CB_4,CB_DATA.F4_CB_5,CB_DATA.F4_CB_6
  Bus Selector20 : BusSelector  OutputSignals=CBStimuli
  Bus Selector36 : BusSelector  OutputSignals=MockEna,ResetAll,GroupSel,F3,F4
  Bus to Vector : BusToVector
  Bus to Vector3 : BusToVector
  Generic_Relay_v2_1 : relay_modbus_lib/Generic_Relay_v2_1  Ts=Ts  relay_settings=[F3(1,:)]
  Generic_Relay_v2_10 : relay_modbus_lib/Generic_Relay_v2_1  Ts=Ts  relay_settings=[F0(3,:)]
  Generic_Relay_v2_11 : relay_modbus_lib/Generic_Relay_v2_1  Ts=Ts  relay_settings=[F3(10,:)]
  Generic_Relay_v2_12 : relay_modbus_lib/Generic_Relay_v2_1  Ts=Ts  relay_settings=[F4(1,:)]
  Generic_Relay_v2_13 : relay_modbus_lib/Generic_Relay_v2_1  Ts=Ts  relay_settings=[F4(2,:)]
  Generic_Relay_v2_14 : relay_modbus_lib/Generic_Relay_v2_1  Ts=Ts  relay_settings=[F4(3,:)]
  Generic_Relay_v2_15 : relay_modbus_lib/Generic_Relay_v2_1  Ts=Ts  relay_settings=[F4(4,:)]
  Generic_Relay_v2_16 : relay_modbus_lib/Generic_Relay_v2_1  Ts=Ts  relay_settings=[F4(5,:)]
  Generic_Relay_v2_17 : relay_modbus_lib/Generic_Relay_v2_1  Ts=Ts  relay_settings=[F4(6,:)]
  Generic_Relay_v2_2 : relay_modbus_lib/Generic_Relay_v2_1  Ts=Ts  relay_settings=[F3(2,:)]
  Generic_Relay_v2_3 : relay_modbus_lib/Generic_Relay_v2_1  Ts=Ts  relay_settings=[F3(3,:)]
  Generic_Relay_v2_4 : relay_modbus_lib/Generic_Relay_v2_1  Ts=Ts  relay_settings=[F3(4,:)]
  Generic_Relay_v2_5 : relay_modbus_lib/Generic_Relay_v2_1  Ts=Ts  relay_settings=[F3(5,:)]
  Generic_Relay_v2_6 : relay_modbus_lib/Generic_Relay_v2_1  Ts=Ts  relay_settings=[F3(6,:)]
  Generic_Relay_v2_7 : relay_modbus_lib/Generic_Relay_v2_1  Ts=Ts  relay_settings=[F3(7,:)]
  Generic_Relay_v2_8 : relay_modbus_lib/Generic_Relay_v2_1  Ts=Ts  relay_settings=[F3(8,:)]
  Generic_Relay_v2_9 : relay_modbus_lib/Generic_Relay_v2_1  Ts=Ts  relay_settings=[F3(9,:)]
  Goto Tag Visibility : GotoTagVisibility  GotoTag=SignalsAll
  Goto Tag Visibility1 : GotoTagVisibility  GotoTag=FastShed
  Memory : Memory
  Memory1 : Memory
  Modbus device : rtio_generic_modbus/Modbus device  conf_name=F3_relay_cfg1.opal  conf_name_mask=F3_relay_cfg1.xls  sample_time=Ts
  Modbus device1 : rtio_generic_modbus/Modbus device  conf_name=F3_relay_cfg2.opal  conf_name_mask=F3_relay_cfg2.xls  sample_time=Ts
  Modbus device10 : rtio_generic_modbus/Modbus device  conf_name=F3_relay_cfg10.opal  conf_name_mask=F3_relay_cfg10.xls  sample_time=Ts
  Modbus device11 : rtio_generic_modbus/Modbus device  conf_name=F4_relay_cfg3.opal  conf_name_mask=F4_relay_cfg3.xls  sample_time=Ts
  Modbus device12 : rtio_generic_modbus/Modbus device  conf_name=F4_relay_cfg4.opal  conf_name_mask=F4_relay_cfg4.xls  sample_time=Ts
  Modbus device13 : rtio_generic_modbus/Modbus device  conf_name=F4_relay_cfg1.opal  conf_name_mask=F4_relay_cfg1.xls  sample_time=Ts
  Modbus device14 : rtio_generic_modbus/Modbus device  conf_name=F4_relay_cfg2.opal  conf_name_mask=F4_relay_cfg2.xls  sample_time=Ts
  Modbus device15 : rtio_generic_modbus/Modbus device  conf_name=F4_relay_cfg5.opal  conf_name_mask=F4_relay_cfg5.xls  sample_time=Ts
  Modbus device16 : rtio_generic_modbus/Modbus device  conf_name=F4_relay_cfg6.opal  conf_name_mask=F4_relay_cfg6.xls  sample_time=Ts
  Modbus device2 : rtio_generic_modbus/Modbus device  conf_name=F3_relay_cfg3.opal  conf_name_mask=F3_relay_cfg3.xls  sample_time=Ts
  Modbus device3 : rtio_generic_modbus/Modbus device  conf_name=F3_relay_cfg4.opal  conf_name_mask=F3_relay_cfg4.xls  sample_time=Ts
  Modbus device4 : rtio_generic_modbus/Modbus device  conf_name=F3_relay_cfg5.opal  conf_name_mask=F3_relay_cfg5.xls  sample_time=Ts
  Modbus device5 : rtio_generic_modbus/Modbus device  conf_name=F3_relay_cfg6.opal  conf_name_mask=F3_relay_cfg6.xls  sample_time=Ts
  Modbus device6 : rtio_generic_modbus/Modbus device  conf_name=F3_relay_cfg7.opal  conf_name_mask=F3_relay_cfg7.xls  sample_time=Ts
  Modbus device7 : rtio_generic_modbus/Modbus device  conf_name=F3_relay_cfg8.opal  conf_name_mask=F3_relay_cfg8.xls  sample_time=Ts
  Modbus device8 : rtio_generic_modbus/Modbus device  conf_name=F3_relay_cfg9.opal  conf_name_mask=F3_relay_cfg9.xls  sample_time=Ts
  Modbus device9 : rtio_generic_modbus/Modbus device  conf_name=F3_relay_cfg_pcc.opal  conf_name_mask=F3_relay_cfg_pcc.xls  sample_time=Ts
  Mux11 : Mux  Inputs=5
  OpComm2 : rtlab/OpComm  nbport=1  groupe_acq=1  subsys_rate=0  st=0  Synchronization=on  Interpolation=on  Threshold=1.0  Missed_Data=off  Sim_Time=off  Samples=off  dynSigOut=off  from_console=0  warning_done=off  writeOpCommFile=off  Offset=off
  OpComm3 : rtlab/OpComm  nbport=3  groupe_acq=1  subsys_rate=0  st=0  Synchronization=on  Interpolation=on  Threshold=1.0  Missed_Data=off  Sim_Time=off  Samples=off  dynSigOut=off  from_console=0  warning_done=off  writeOpCommFile=off  Offset=off
  SelectMockup : relay_modbus_lib/SelectMockup  sigID=4  sigN=17
  SelectMockup1 : relay_modbus_lib/SelectMockup  sigID=3  sigN=17
  SelectMockup10 : relay_modbus_lib/SelectMockup  sigID=10  sigN=17
  SelectMockup11 : relay_modbus_lib/SelectMockup  sigID=13  sigN=17
  SelectMockup12 : relay_modbus_lib/SelectMockup  sigID=16  sigN=17
  SelectMockup13 : relay_modbus_lib/SelectMockup  sigID=12  sigN=17
  SelectMockup14 : relay_modbus_lib/SelectMockup  sigID=17  sigN=17
  SelectMockup15 : relay_modbus_lib/SelectMockup  sigID=15  sigN=17
  SelectMockup16 : relay_modbus_lib/SelectMockup  sigID=14  sigN=17
  SelectMockup2 : relay_modbus_lib/SelectMockup  sigID=2  sigN=17
  SelectMockup3 : relay_modbus_lib/SelectMockup  sigID=1  sigN=17
  SelectMockup4 : relay_modbus_lib/SelectMockup  sigID=5  sigN=17
  SelectMockup5 : relay_modbus_lib/SelectMockup  sigID=6  sigN=17
  SelectMockup6 : relay_modbus_lib/SelectMockup  sigID=7  sigN=17
  SelectMockup7 : relay_modbus_lib/SelectMockup  sigID=8  sigN=17
  SelectMockup8 : relay_modbus_lib/SelectMockup  sigID=9  sigN=17
  SelectMockup9 : relay_modbus_lib/SelectMockup  sigID=11  sigN=17
  Subsystem : Subsystem
  F3_RELAY _OUT : Outport
  F4_RELAY _OUT : Outport  Port=2
  tag scope: FastShed=scoped, SignalsAll=scoped
  wires:
  Bus to Vector3/1 -> Mux11/5
  Bus Selector36/5 -> Bus to Vector3/1  "<F4>"
  Bus Creator2/1 -> Bus Creator3/7  "F4_CB_CTRL"
  SelectMockup14/2 -> Bus Creator2/6
  SelectMockup12/2 -> Bus Creator2/5
  SelectMockup15/2 -> Bus Creator2/4
  SelectMockup16/2 -> Bus Creator2/3
  SelectMockup11/2 -> Bus Creator2/2
  SelectMockup13/2 -> Bus Creator2/1
  OpComm3/3 -> Bus Selector2/1
  Generic_Relay_v2_12/2 -> Modbus device13/1
  F4_MS_IN/1 -> OpComm3/3
  Bus Selector2/1 -> Generic_Relay_v2_12/1  "<F4_CB_1>"
  Bus Selector2/2 -> Generic_Relay_v2_13/1  "<F4_CB_2>"
  Bus Selector2/3 -> Generic_Relay_v2_14/1  "<F4_CB_3>"
  Bus Selector2/4 -> Generic_Relay_v2_15/1  "<F4_CB_4>"
  Bus Selector2/5 -> Generic_Relay_v2_16/1  "<F4_CB_5>"
  Bus Selector2/6 -> Generic_Relay_v2_17/1  "<F4_CB_6>"
  Generic_Relay_v2_12/1 -> Bus Creator3/1  "F4_CB_1"
  Generic_Relay_v2_13/1 -> Bus Creator3/2  "F4_CB_2"
  Generic_Relay_v2_14/1 -> Bus Creator3/3  "F4_CB_3"
  Generic_Relay_v2_15/1 -> Bus Creator3/4  "F4_CB_4"
  Generic_Relay_v2_16/1 -> Bus Creator3/5  "F4_CB_5"
  Generic_Relay_v2_17/1 -> Bus Creator3/6  "F4_CB_6"
  Bus Creator3/1 -> Memory1/1
  Memory1/1 -> F4_RELAY _OUT/1
  Generic_Relay_v2_14/2 -> Modbus device11/1
  Generic_Relay_v2_15/2 -> Modbus device12/1
  Modbus device13/1 -> SelectMockup13/1
  SelectMockup13/1 -> Generic_Relay_v2_12/2
  Generic_Relay_v2_13/2 -> Modbus device14/1
  Modbus device14/1 -> SelectMockup11/1
  SelectMockup11/1 -> Generic_Relay_v2_13/2
  Generic_Relay_v2_16/2 -> Modbus device15/1
  Modbus device15/1 -> SelectMockup12/1
  SelectMockup12/1 -> Generic_Relay_v2_16/2
  Generic_Relay_v2_17/2 -> Modbus device16/1
  Modbus device16/1 -> SelectMockup14/1
  SelectMockup14/1 -> Generic_Relay_v2_17/2
  Modbus device12/1 -> SelectMockup15/1
  SelectMockup15/1 -> Generic_Relay_v2_15/2
  SelectMockup16/1 -> Generic_Relay_v2_14/2
  Modbus device11/1 -> SelectMockup16/1
  Bus Creator1/1 -> Bus Creator6/12  "F3_CB_CTRL"
  SelectMockup9/2 -> Bus Creator1/11
  SelectMockup10/2 -> Bus Creator1/10
  SelectMockup8/2 -> Bus Creator1/9
  SelectMockup7/2 -> Bus Creator1/8
  SelectMockup6/2 -> Bus Creator1/7
  SelectMockup5/2 -> Bus Creator1/6
  SelectMockup4/2 -> Bus Creator1/5
  SelectMockup/2 -> Bus Creator1/4
  SelectMockup1/2 -> Bus Creator1/3
  SelectMockup2/2 -> Bus Creator1/2
  SelectMockup3/2 -> Bus Creator1/1
  Subsystem/1(vect) -> [FastShed]
  OpComm3/2 -> Subsystem/1(bus)
  GOOSE_TRIP/1 -> OpComm3/2
  Bus Selector1/11 -> Generic_Relay_v2_10/1  "<F3_PCC>"
  Modbus device10/1 -> SelectMockup10/1
  SelectMockup10/1 -> Generic_Relay_v2_11/2
  Generic_Relay_v2_11/2 -> Modbus device10/1
  Generic_Relay_v2_11/1 -> Bus Creator6/10  "F3_CB_10"
  Modbus device2/1 -> SelectMockup1/1
  Modbus device/1 -> SelectMockup3/1
  Modbus device1/1 -> SelectMockup2/1
  Modbus device3/1 -> SelectMockup/1
  Modbus device4/1 -> SelectMockup4/1
  Modbus device5/1 -> SelectMockup5/1
  Modbus device6/1 -> SelectMockup6/1
  Modbus device7/1 -> SelectMockup7/1
  Modbus device8/1 -> SelectMockup8/1
  Modbus device9/1 -> SelectMockup9/1
  Mux11/1 -> [SignalsAll]
  Bus Selector36/2 -> Mux11/2  "<ResetAll>"
  Bus Selector36/3 -> Mux11/3  "<GroupSel>"
  Bus to Vector/1 -> Mux11/4
  Bus Selector36/1 -> Mux11/1  "<MockEna>"
  Bus Selector36/4 -> Bus to Vector/1  "<F3>"
  Bus Selector20/1 -> Bus Selector36/1  "<CBStimuli>"
  OpComm2/1 -> Bus Selector20/1
  SC_CMD/1 -> OpComm2/1
  Bus Selector1/10 -> Generic_Relay_v2_11/1  "<F3_CB_10>"
  SelectMockup9/1 -> Generic_Relay_v2_10/2
  Generic_Relay_v2_10/2 -> Modbus device9/1
  Generic_Relay_v2_10/1 -> Bus Creator6/11  "F3_PCC"
  Memory/1 -> F3_RELAY _OUT/1
  Bus Selector1/8 -> Generic_Relay_v2_8/1  "<F3_CB_8>"
  Bus Selector1/9 -> Generic_Relay_v2_9/1  "<F3_CB_9>"
  Generic_Relay_v2_9/1 -> Bus Creator6/9  "F3_CB_9"
  Generic_Relay_v2_8/1 -> Bus Creator6/8  "F3_CB_8"
  SelectMockup8/1 -> Generic_Relay_v2_9/2
  Generic_Relay_v2_9/2 -> Modbus device8/1
  Generic_Relay_v2_8/2 -> Modbus device7/1
  SelectMockup7/1 -> Generic_Relay_v2_8/2
  Bus Creator6/1 -> Memory/1
  Generic_Relay_v2_7/1 -> Bus Creator6/7  "F3_CB_7"
  Generic_Relay_v2_6/1 -> Bus Creator6/6  "F3_CB_6"
  Generic_Relay_v2_5/1 -> Bus Creator6/5  "F3_CB_5"
  Generic_Relay_v2_4/1 -> Bus Creator6/4  "F3_CB_4"
  Generic_Relay_v2_3/1 -> Bus Creator6/3  "F3_CB_3"
  Generic_Relay_v2_2/1 -> Bus Creator6/2  "F3_CB_2"
  Generic_Relay_v2_1/1 -> Bus Creator6/1  "F3_CB_1"
  Bus Selector1/7 -> Generic_Relay_v2_7/1  "<F3_CB_7>"
  Bus Selector1/6 -> Generic_Relay_v2_6/1  "<F3_CB_6>"
  Bus Selector1/5 -> Generic_Relay_v2_5/1  "<F3_CB_5>"
  Bus Selector1/4 -> Generic_Relay_v2_4/1  "<F3_CB_4>"
  Bus Selector1/3 -> Generic_Relay_v2_3/1  "<F3_CB_3>"
  Bus Selector1/2 -> Generic_Relay_v2_2/1  "<F3_CB_2>"
  Bus Selector1/1 -> Generic_Relay_v2_1/1  "<F3_CB_1>"
  F3_MS_IN/1 -> OpComm3/1
  SelectMockup6/1 -> Generic_Relay_v2_7/2
  Generic_Relay_v2_7/2 -> Modbus device6/1
  Generic_Relay_v2_6/2 -> Modbus device5/1
  SelectMockup5/1 -> Generic_Relay_v2_6/2
  SelectMockup4/1 -> Generic_Relay_v2_5/2
  Generic_Relay_v2_5/2 -> Modbus device4/1
  SelectMockup/1 -> Generic_Relay_v2_4/2
  Generic_Relay_v2_4/2 -> Modbus device3/1
  Generic_Relay_v2_3/2 -> Modbus device2/1
  SelectMockup1/1 -> Generic_Relay_v2_3/2
  SelectMockup2/1 -> Generic_Relay_v2_2/2
  Generic_Relay_v2_2/2 -> Modbus device1/1
  SelectMockup3/1 -> Generic_Relay_v2_1/2
  Generic_Relay_v2_1/2 -> Modbus device/1
  OpComm3/1 -> Bus Selector1/1
